simulink subsystem "Reductor"  (R2022b)
settings: Solver=VariableStepAuto  StartTime=0.0  StopTime=10.0  RelTol=1e-3
undefined symbols (not defined in the file): ProjectExample
settings Model: Creator=Ilya_Andriyanov  LastModifiedBy=user

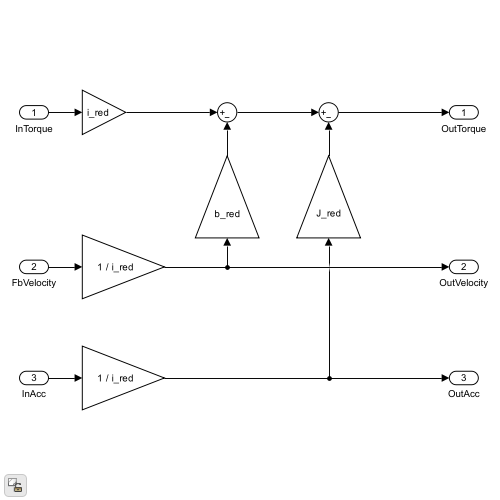
[thumbnail: Simulink's stored preview of the top-level diagram]
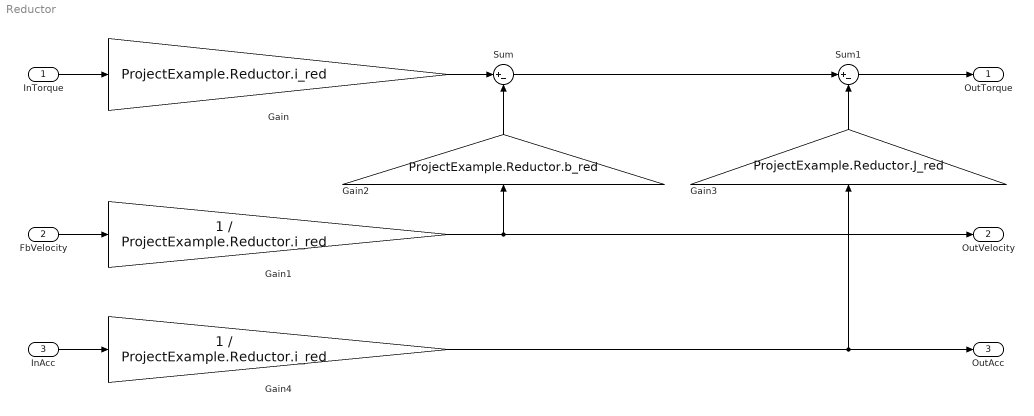
== system Reductor ==
  InTorque : Inport
  FbVelocity : Inport  Port=2
  InAcc : Inport  Port=3
  Gain : Gain  Gain=ProjectExample.Reductor.i_red
  Gain1 : Gain  Gain=1 / ProjectExample.Reductor.i_red
  Gain2 : Gain  Gain=ProjectExample.Reductor.b_red
  Gain3 : Gain  Gain=ProjectExample.Reductor.J_red
  Gain4 : Gain  Gain=1 / ProjectExample.Reductor.i_red
  Sum : Sum  Inputs=|+-
  Sum1 : Sum  Inputs=|+-
  OutTorque : Outport
  OutVelocity : Outport  Port=2
  OutAcc : Outport  Port=3
  wires:
  InTorque/1 -> Gain/1
  Gain/1 -> Sum/1
  Sum/1 -> Sum1/1
  Sum1/1 -> OutTorque/1
  FbVelocity/1 -> Gain1/1
  Gain1/1 -> OutVelocity/1, Gain2/1
  Gain2/1 -> Sum/2
  InAcc/1 -> Gain4/1
  Gain3/1 -> Sum1/2
  Gain4/1 -> Gain3/1, OutAcc/1
